simulink model "CHE360_Hw5_Q1"  (R2018a)
settings: Solver=VariableStepAuto  StartTime=0.0  StopTime=2  RelTol=1e-3
settings Model: Creator=kr27867  LastModifiedBy=kr27867

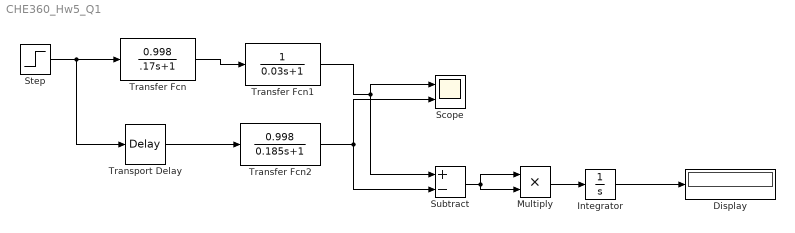
== system CHE360_Hw5_Q1 ==
  Display : Display
  Integrator : Integrator
  Multiply : Product
  Scope : Scope  NumInputPorts=2
  Step : Step  SampleTime=0
  Subtract : Sum  Inputs=+-
  Transfer Fcn : TransferFcn  Numerator=[0.998]  Denominator=[.17 1]
  Transfer Fcn1 : TransferFcn  Denominator=[0.03 1]
  Transfer Fcn2 : TransferFcn  Numerator=[0.998]  Denominator=[0.185 1]
  Transport Delay : TransportDelay  DelayTime=0.015
  wires:
  Step/1 -> Transport Delay/1, Transfer Fcn/1
  Transfer Fcn/1 -> Transfer Fcn1/1
  Transfer Fcn1/1 -> Subtract/1, Scope/1
  Transport Delay/1 -> Transfer Fcn2/1
  Transfer Fcn2/1 -> Subtract/2, Scope/2
  Subtract/1 -> Multiply/2, Multiply/1
  Multiply/1 -> Integrator/1
  Integrator/1 -> Display/1
